simulink model "namrata_lab7_3_1"  (R2018b)
settings: Solver=VariableStepAuto  StartTime=0.0  StopTime=10.0  RelTol=1e-3
settings Model: Creator=student  LastModifiedBy=student

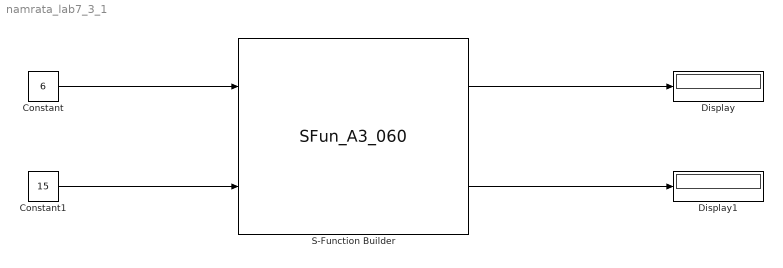
== system namrata_lab7_3_1 ==
  Constant : Constant  Value=6
  Constant1 : Constant  Value=15
  Display : Display
  Display1 : Display
  S-Function Builder : S-Function  InitFcn=try, set_param(gcb,'FunctionName','SFun_A3_060'), end  FunctionName=SFun_A3_060  SFunctionModules=SFun_A3_060_wrapper  SFunctionDeploymentMode=off  EnableBusSupport=off  mask(S-Function Builder){}
      mask help: Simulink:masks:SFunctionBuilder_MD
      mask init:
      | val = [[.9  0.75 0.75 1 1 .9 .9 1]',[1 1 0.75 0.75 .9 .9 1 .9]'];try , sys = get_param(gcb,'SfunBuilderFcnName');if isempty(sys), sys = get_param(gcb,'FunctionName'); end,catch, sys = get_param(gcb,'FunctionName'); end
      settings: CopyFcn=set_param(gcbh,'LinkStatus','none')  PreSaveFcn=try, set_param(gcb,'FunctionName','SFun_A3_060'), end  OpenFcn=sfunctionwizard(gcbh)
      mask Display: image('Lighthouse.jpg')
  wires:
  Constant/1 -> S-Function Builder/1
  Constant1/1 -> S-Function Builder/2
  S-Function Builder/1 -> Display/1
  S-Function Builder/2 -> Display1/1
